simulink model "doc_ortho"  (Simulink 6.0)
settings: Solver=FixedStepDiscrete  StartTime=0.0  StopTime=127  RelTol=1e-3
undefined symbols (not defined in the file): slcm
libraries: commseqgen2 x3, dspsnks4 x3
settings Model: Creator=akansal  LastModifiedBy=agaltman  ProdHWDeviceType=Specified
settings DataIOCC: SignalLoggingName=sigsOut
settings OptimizationCC: BooleanDataType=off  MultiInstanced=off
settings FormatCC: IgnoreBidirectionalLines=off
settings HardwareCC: ProdHWDeviceType=Specified
settings CodeAppCC: FileBanners=off  CustomSymbols=off  MangleLength=5
settings GRTTargetCC: TargetFcnLib=iso_c_tmw.mat  IsERTTarget=off

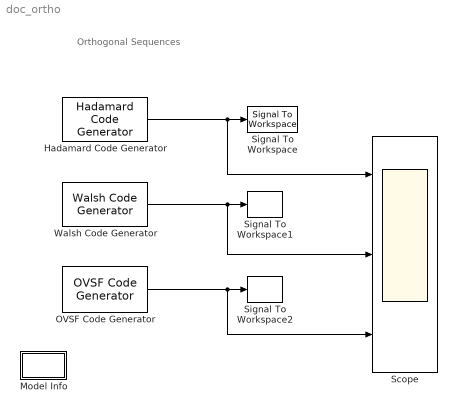
== system doc_ortho ==
  note: Orthogonal Sequences
  Hadamard Code Generator : commseqgen2/Hadamard Code Generator  length=64  index=31  ts=1  frameBased=off  sampPerFrame=1
  Model Info : Subsystem  LoadFcn=slcm LoadBlock;  InitFcn=slcm('UpdateAllCMBlocksInThisModelInit')  mask(CMBlock){InitialSaveTempField=, InitialBlockCM=None, BlockCM=None, Frame=on, SaveTempField=, DisplayStringWithTags=Info, MaskDisplayString=Info, HorizontalTextAlignment=Center, LeftAlignmentValue=0.5, SourceBlockDiagram=doc_ortho, TagMaxNumber=20, CMTag1=, CMTag2=, CMTag3=, CMTag4=, CMTag5=, CMTag6=, CMTag7=, CMTag8=, CMTag9=, CMTag10=, CMTag11=, CMTag12=, CMTag13=, CMTag14=, CMTag15=, CMTag16=, CMTag17=, CMTag18=, CMTag19=, CMTag20=}
      mask help: This block allows revision control information to be displayed within the model.
      settings: CopyFcn=slcm CopyBlock;  DeleteFcn=slcm Cancel;  PostSaveFcn=slcm('UpdateAllCMBlocksInThisModel')  NameChangeFcn=slcm Rename;  OpenFcn=commdemohelp;
      mask Display: text(str2num(LeftAlignmentValue), 0.5, MaskDisplayString, 'HorizontalAlignment', HorizontalTextAlignment)
  OVSF Code Generator : commseqgen2/OVSF Code Generator  spreadFact=64  index=31  ts=1  frameBased=off  sampPerFrame=1
  Scope : Scope  NumInputPorts=3
      settings: YMin=-1.5~-1.5~-1.5  YMax=1.5~1.5~1.5
  Signal To Workspace : dspsnks4/Signal To Workspace  VariableName=had  FrameMode=Concatenate frames (2-D array)
  Signal To Workspace1 : dspsnks4/Signal To Workspace  VariableName=walsh  FrameMode=Concatenate frames (2-D array)
  Signal To Workspace2 : dspsnks4/Signal To Workspace  VariableName=ovsf  FrameMode=Concatenate frames (2-D array)
  Walsh Code Generator : commseqgen2/Walsh Code Generator  length=64  index=31  ts=1  frameBased=off  sampPerFrame=1
  wires:
  Hadamard Code Generator/1 -> Signal To Workspace/1, Scope/1
  Walsh Code Generator/1 -> Signal To Workspace1/1, Scope/2
  OVSF Code Generator/1 -> Signal To Workspace2/1, Scope/3

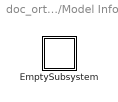
== system doc_ortho/Model Info ==
  EmptySubsystem : Subsystem

== system doc_ortho/Model Info/EmptySubsystem ==
